simulink model "GA25_370_130RPM_model"  (R2025b)
settings: Solver=VariableStepAuto  StartTime=0.0  StopTime=10.0  RelTol=1e-3
undefined symbols (not defined in the file or in its folder): b, J, kb, Kma, La, Ra
settings Model: Creator=tarek  LastModifiedBy=tarek

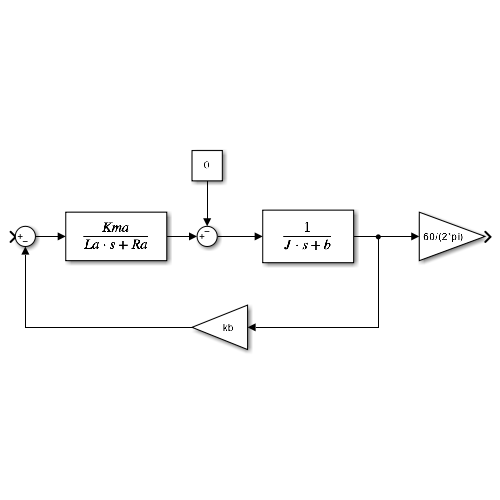
[thumbnail: Simulink's stored preview of the top-level diagram]
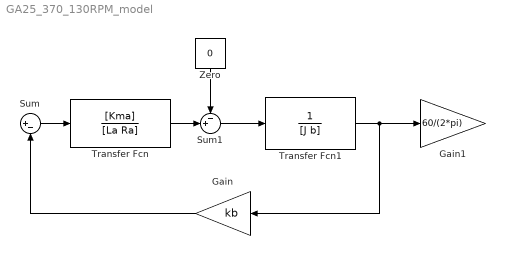
== system GA25_370_130RPM_model ==
  Gain : Gain  Gain=kb
  Gain1 : Gain  Gain=60/(2*pi)
  Sum : Sum  Inputs=|+-
  Sum1 : Sum  Inputs=-+|
  Transfer Fcn : TransferFcn  Numerator=[Kma]  Denominator=[La Ra]
  Transfer Fcn1 : TransferFcn  Denominator=[J b]
  Zero : Constant  Value=0  OutDataTypeStr=Inherit: Inherit via back propagation
  wires:
  Transfer Fcn/1 -> Sum1/2
  Zero/1 -> Sum1/1
  Sum1/1 -> Transfer Fcn1/1
  Gain/1 -> Sum/2
  Transfer Fcn1/1 -> Gain1/1, Gain/1
  Sum/1 -> Transfer Fcn/1
